simulink model "bai12"  (R2022b)
settings: Solver=VariableStepAuto  StartTime=0.0  StopTime=20.0  RelTol=1e-8
values from neighbouring files (symbols this model uses):
  k0 = -8    [bai21111.m]
  k1 = -1    [bai21111.m]
settings Model: Creator=ASUS  LastModifiedBy=admin

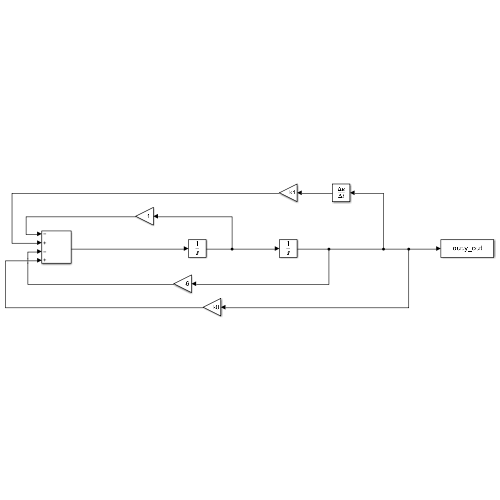
[thumbnail: Simulink's stored preview of the top-level diagram]
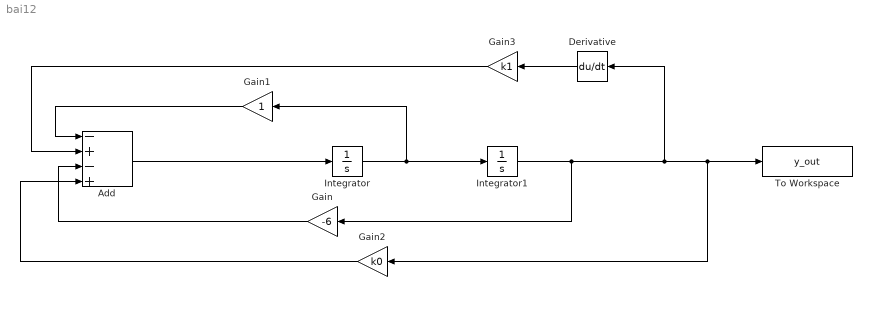
== system bai12 ==
  Add : Sum  Inputs=-+-+
  Derivative : Derivative
  Gain : Gain  Gain=-6
  Gain1 : Gain
  Gain2 : Gain  Gain=k0
  Gain3 : Gain  Gain=k1
  Integrator : Integrator  InitialCondition=5
  Integrator1 : Integrator
  To Workspace : ToWorkspace  VariableName=y_out  SaveFormat=Structure With Time  SampleTime=-1
  wires:
  Gain3/1 -> Add/2
  Add/1 -> Integrator/1
  Integrator/1 -> Gain1/1, Integrator1/1
  Integrator1/1 -> Derivative/1, Gain2/1, To Workspace/1, Gain/1
  Gain/1 -> Add/3
  Gain1/1 -> Add/1
  Gain2/1 -> Add/4
  Derivative/1 -> Gain3/1
